simulink model "EJ2P2"  (R2019a)
settings: Solver=ode3  StartTime=0.0  StopTime=10.0  FixedStep=0.01  RelTol=1e-3
undefined symbols (not defined in the file or in its folder): DiscIntNeverNeededParam
libraries: simulink x1
settings Model: EnablePacing=on  Creator=mrblissfulgrin  LastModifiedBy=mrblissfulgrin
settings DataIOCC: ReturnWorkspaceOutputs=off

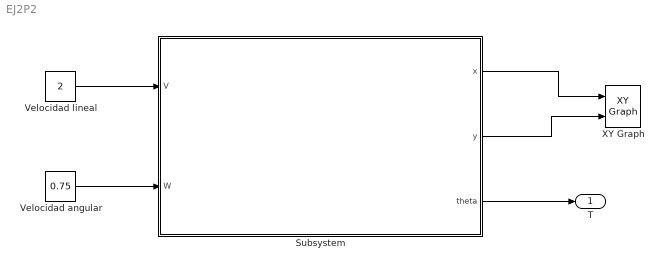
== system EJ2P2 ==
  Subsystem : Subsystem
  Velocidad angular : Constant  Value=0.75  SampleTime=0.01
  Velocidad lineal : Constant  Value=2  SampleTime=0.01
  XY Graph : simulink/Sinks/XY Graph  xmin=-5  xmax=5  ymin=-5  ymax=5  st=0.01
  T : Outport
  wires:
  Velocidad lineal/1 -> Subsystem/1(V)
  Subsystem/1(x) -> XY Graph/1
  Subsystem/2(y) -> XY Graph/2
  Subsystem/3(theta) -> T/1
  Velocidad angular/1 -> Subsystem/2(W)

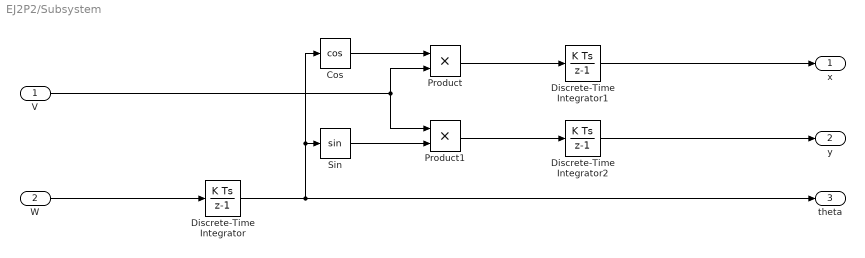
== system EJ2P2/Subsystem ==
  V : Inport
  W : Inport  Port=2
  Cos : Trigonometry  Operator=cos
  Discrete-Time Integrator : DiscreteIntegrator  InitialCondition=30*pi/180  SampleTime=0.01  ICPrevOutput=DiscIntNeverNeededParam  ICPrevScaledInput=DiscIntNeverNeededParam
  Discrete-Time Integrator1 : DiscreteIntegrator  InitialCondition=-4  SampleTime=0.01  ICPrevOutput=DiscIntNeverNeededParam  ICPrevScaledInput=DiscIntNeverNeededParam
  Discrete-Time Integrator2 : DiscreteIntegrator  InitialCondition=-4  SampleTime=0.01  ICPrevOutput=DiscIntNeverNeededParam  ICPrevScaledInput=DiscIntNeverNeededParam
  Product : Product
  Product1 : Product
  Sin : Trigonometry
  x : Outport
  y : Outport  Port=2
  theta : Outport  Port=3
  wires:
  Discrete-Time Integrator2/1 -> y/1
  Product1/1 -> Discrete-Time Integrator2/1
  Cos/1 -> Product/1
  Sin/1 -> Product1/2
  W/1 -> Discrete-Time Integrator/1
  Discrete-Time Integrator1/1 -> x/1
  Product/1 -> Discrete-Time Integrator1/1
  V/1 -> Product/2, Product1/1
  Discrete-Time Integrator/1 -> theta/1, Sin/1, Cos/1
